simulink library "Input_Fluid"  (Simulink 8.2)
settings: Solver=ode45  StartTime=0.0  StopTime=10.0  RelTol=1e-3
settings Model: Creator=lena.frank  LastModifiedBy=drhf

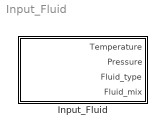
== system Input_Fluid ==
  Input_Fluid : Subsystem  mask(Input_Fluid){fluid=Water, T=[10:10:50], p=1e5, x=0.005}
      mask prompts: fluid "Fluid type"; T "temperature (scalar or vector) [°C]"; p "pressure [Pa]"; x "Fluid Mix"
      mask help:
      | FLUID            FLUID MIX
      | water          vapourcontent in the 2-phase region
      | air               (kg water) / (kg dry air)
      | cotton oil       -
      | silicone oil     -
      | water-glycol   volume partition [0..1] of propylen glycol
      mask Help: web(fullfile(path_carnot('help'),'input_material.html'),'-helpbrowser')
      mask TypeOptions fluid: Water | Air | Cotton Oil | Silicone Oil | Water-Glycol Mix | Tyfocor LS | Water (Constant 20°C) | Air (dry+ constant 20°C)

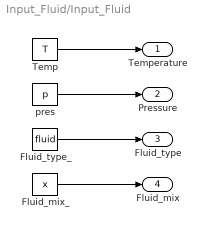
== system Input_Fluid/Input_Fluid ==
  Fluid_mix_ : Constant  Value=x
  Fluid_type_ : Constant  Value=fluid
  Temp : Constant  Value=T
  pres : Constant  Value=p
  Temperature : Outport
  Pressure : Outport  Port=2
  Fluid_type : Outport  Port=3
  Fluid_mix : Outport  Port=4
  wires:
  Fluid_mix_/1 -> Fluid_mix/1
  Fluid_type_/1 -> Fluid_type/1
  Temp/1 -> Temperature/1
  pres/1 -> Pressure/1
